simulink model "AUV_sim_loopshaping"  (R2016b)
settings: Solver=ode45  StartTime=0.0  StopTime=100  RelTol=1e-3  EnableMultiTasking=on
InitFcn:
  | param
undefined symbols (not defined in the file or in its folder): AUV_ctrl_loop, P
settings Model: Creator=beard  LastModifiedBy=Jacob
settings DataIOCC: LimitDataPoints=on  SaveFormat=Array  SignalLoggingSaveFormat=ModelDataLogs
settings OptimizationCC: ExpressionDepthLimit=2147483647  InitFltsAndDblsToZero=on  LifeSpan=inf
settings DebuggingCC: UnderspecifiedInitializationDetection=Classic  MergeDetectMultiDrivingBlocksExec=none  SolverPrmCheckMsg=warning  FcnCallInpInsideContextMsg=warning  StateNameClashWarn=warning  SFUnexpectedBacktrackingDiag=warning  SFNoUnconditionalDefaultTransitionDiag=warning  SFExecutionAtInitializationDiag=none
settings HardwareCC: ProdBitPerPointer=32  ProdBitPerSizeT=32  ProdBitPerPtrDiffT=32  ProdLargestAtomicFloat=None  ProdIntDivRoundTo=Undefined  ProdEndianess=Unspecified  ProdWordSize=32  ProdHWDeviceType=32-bit Generic
settings ModelReferenceCC: PropagateSignalLabelsOutOfModel=off
settings GRTTargetCC: TargetLangStandard=C89/C90 (ANSI)  GeneratePreprocessorConditionals=Disable all  CombineOutputUpdateFcns=off  GRTInterface=on
settings ConfigComp: CovMetricSettings=dw  CovHtmlReporting=on  CovSaveCumulativeToWorkspaceVar=on  CovSaveSingleToWorkspaceVar=on  CovExternalEMLEnable=off

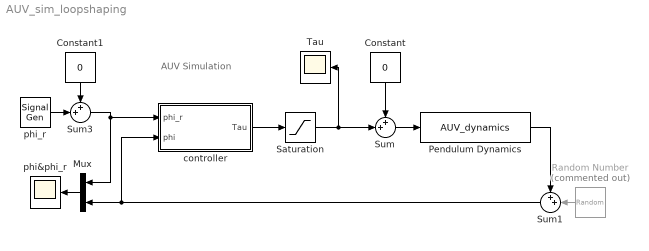
== system AUV_sim_loopshaping ==
  note: AUV Simulation
  Constant : Constant  Value=0
  Constant1 : Constant  Value=0
  Mux : Mux  Inputs=2
  Pendulum Dynamics : S-Function  FunctionName=AUV_dynamics  Parameters=P  SFunctionDeploymentMode=off  EnableBusSupport=off
  Random Number : RandomNumber  Commented=on  Variance=.001^2  SampleTime=P.Ts
  Saturation : Saturate  UpperLimit=P.Taumax  LowerLimit=-P.Taumax
  Sum : Sum  Inputs=++|
  Sum1 : Sum  Inputs=++|
  Sum3 : Sum  Inputs=++|
  Tau : Scope
  controller : Subsystem
  phi&phi_r : Scope
  phi_r : SignalGenerator  WaveForm=square  Amplitude=0.5  Frequency=.02
  wires:
  Pendulum Dynamics/1 -> Sum1/1
  controller/1(Tau) -> Saturation/1
  Saturation/1 -> Sum/2, Tau/1
  Mux/1 -> phi&phi_r/1
  Sum/1 -> Pendulum Dynamics/1
  Sum1/1 -> controller/2(phi), Mux/2
  Random Number/1 -> Sum1/2
  Constant/1 -> Sum/1
  phi_r/1 -> Sum3/2
  Sum3/1 -> Mux/1, controller/1(phi_r)
  Constant1/1 -> Sum3/1

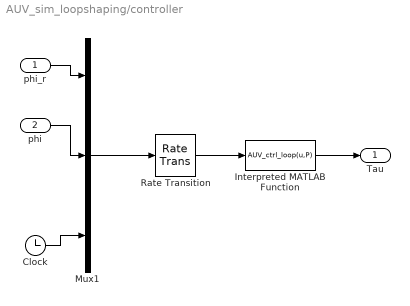
== system AUV_sim_loopshaping/controller ==
  phi_r : Inport
  phi : Inport  Port=2
  Clock : Clock
  Interpreted MATLAB Function : MATLABFcn  MATLABFcn=AUV_ctrl_loop(u,P)  OutputDimensions=1
  Mux1 : Mux  Inputs=3
  Rate Transition : RateTransition  OutPortSampleTime=P.Ts
  Tau : Outport
  wires:
  Mux1/1 -> Rate Transition/1
  phi_r/1 -> Mux1/1
  Rate Transition/1 -> Interpreted MATLAB Function/1
  phi/1 -> Mux1/2
  Interpreted MATLAB Function/1 -> Tau/1
  Clock/1 -> Mux1/3
